simulink model "SG__MDL_IO334"  (R2022b)
settings: Solver=FixedStepAuto  StartTime=0.0  StopTime=Inf  RelTol=1e-3  EnableMultiTasking=on
model workspace (MAT data in the model file):
  a = 0.28
  ff = 1200
  fi = 150
  tmax = 40
libraries: simulink x6, dspsigops x5, hdlsllib x2, slrealtimeloglib x1, SG_library x1, dspsrcs4 x1
settings Model: SimulationMode=external  Creator=padlewsk  LastModifiedBy=padlewsk
settings SolverCC: ConcurrentTasks=on  AlgebraicLoopSolver=TrustRegion  PositivePriorityOrder=on  AutoInsertRateTranBlk=on
settings DataIOCC: SaveFormat=StructureWithTime
settings OptimizationCC: BlockReduction=off  OptimizeBlockIOStorage=off
settings DebuggingCC: TasksWithSamePriorityMsg=none  UnconnectedInputMsg=warning  UnconnectedOutputMsg=warning  UnconnectedLineMsg=warning
settings HardwareCC: ProdBitPerLong=64  ProdLongLongMode=on  ProdHWDeviceType=Intel->x86-64 (Linux 64)
settings ModelReferenceCC: EnableRefExpFcnMdlSchedulingChecks=on
settings RTWCC: Description=Simulink Real-Time  SystemTargetFile=slrealtime.tlc  TemplateMakefile=slrealtime_default_tmf  Toolchain=Simulink Real-Time Toolchain  BuildConfiguration=Faster Runs  CodeExecutionProfiling=on  TargetLang=C++

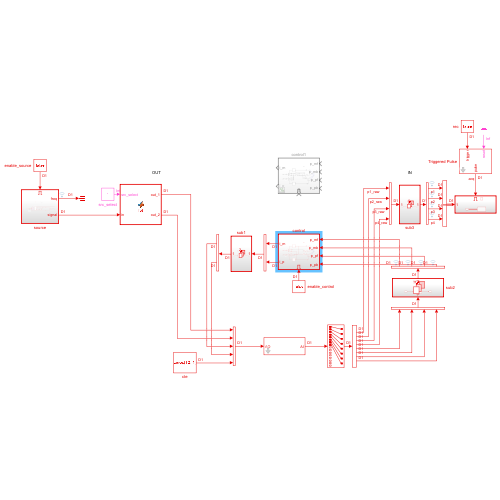
[thumbnail: Simulink's stored preview of the top-level diagram]
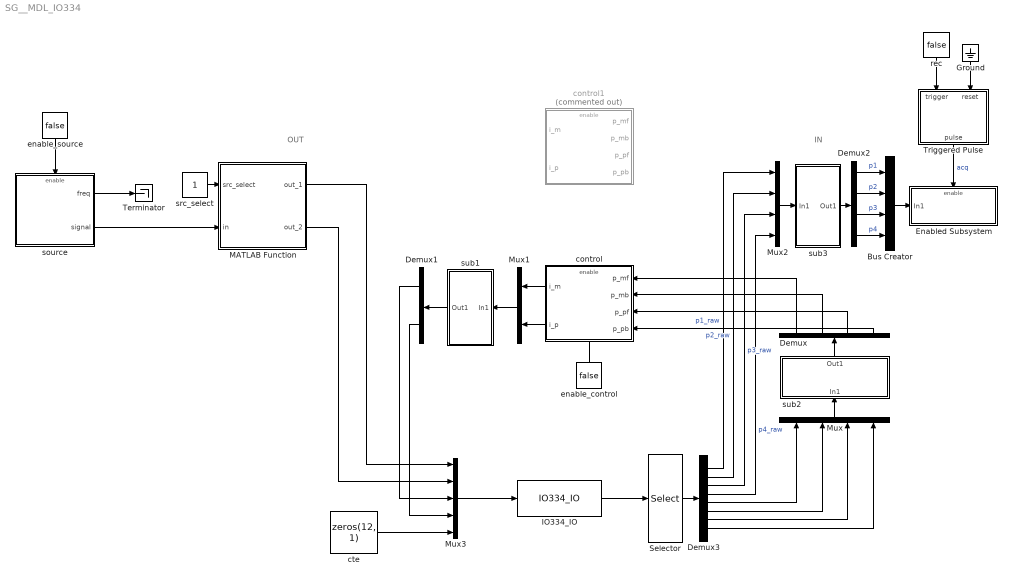
== system SG__MDL_IO334 ==
  note: IN
  note: OUT
  Bus Creator : BusCreator  Inputs=4
  Demux : Demux
  Demux1 : Demux  Outputs=2
  Demux2 : Demux
  Demux3 : Demux  Outputs=8
  Enabled Subsystem : Subsystem  TreatAsAtomicUnit=on
  Ground : Ground
  IO334_IO : SG_library/Built elements/IO334_IO  ts=2.5e-05  OutputRange=Auto (same as ADC)
  MATLAB Function : MATLAB Function  TreatAsAtomicUnit=on
  Mux : Mux
  Mux1 : Mux  Inputs=2
  Mux2 : Mux
  Mux3 : Mux  Inputs=5
  Selector : Selector  InputPortWidth=16  IndexOptions=Index vector (dialog)  Indices=1:8  OutputSizes=1
  Terminator : Terminator
  Triggered Pulse : Subsystem  mask(Triggered Pulse){N=4}
      mask prompts: N "Length (N samples)"
      mask help: Generates a single pulse of N samples length
  control : Subsystem
  control1 : Subsystem  Commented=on
  cte : Constant  Value=zeros(12, 1)  SampleTime=-1
  enable_control : Constant  Value=false  SampleTime=-1
  enable_source : Constant  Value=false  SampleTime=-1
  rec : Constant  Value=false  SampleTime=-1
  source : Subsystem  TreatAsAtomicUnit=on
  src_select : Constant
  sub1 : Subsystem  TreatAsAtomicUnit=on
  sub2 : Subsystem  TreatAsAtomicUnit=on
  sub3 : Subsystem  TreatAsAtomicUnit=on
  wires:
  enable_source/1 -> source/Enable
  Ground/1 -> Triggered Pulse/2(reset)
  rec/1 -> Triggered Pulse/1(trigger)
  Bus Creator/1 -> Enabled Subsystem/1(In1)
  source/1(freq) -> Terminator/1
  source/2(signal) -> MATLAB Function/2(in)
  src_select/1 -> MATLAB Function/1(src_select)
  Mux/1 -> sub2/1(In1)
  sub2/1(Out1) -> Demux/1
  Mux1/1 -> sub1/1(In1)
  sub1/1(Out1) -> Demux1/1
  sub3/1(Out1) -> Demux2/1
  Mux2/1 -> sub3/1(In1)
  Demux3/1 -> Mux2/1  "p1_raw"
  Demux3/2 -> Mux2/2  "p2_raw"
  Demux3/3 -> Mux2/3  "p3_raw"
  Demux3/4 -> Mux2/4  "p4_raw"
  Demux2/2 -> Bus Creator/2  "p2"
  Demux2/1 -> Bus Creator/1  "p1"
  Demux2/3 -> Bus Creator/3  "p3"
  Demux2/4 -> Bus Creator/4  "p4"
  control/1(i_m) -> Mux1/1
  control/2(i_p) -> Mux1/2
  enable_control/1 -> control/Enable
  Demux/1 -> control/1(p_mf)
  Demux/2 -> control/2(p_mb)
  Demux/3 -> control/3(p_pf)
  Demux/4 -> control/4(p_pb)
  IO334_IO/1 -> Selector/1
  Mux3/1 -> IO334_IO/1
  Selector/1 -> Demux3/1
  Demux3/5 -> Mux/1
  Demux3/6 -> Mux/2
  Demux3/7 -> Mux/3
  Demux3/8 -> Mux/4
  cte/1 -> Mux3/5
  Demux1/1 -> Mux3/3
  Demux1/2 -> Mux3/4
  MATLAB Function/2(out_2) -> Mux3/2
  MATLAB Function/1(out_1) -> Mux3/1
  Triggered Pulse/1(pulse) -> Enabled Subsystem/Enable  "acq"

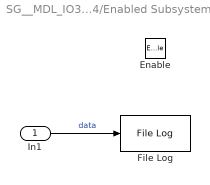
== system SG__MDL_IO334/Enabled Subsystem ==
  In1 : Inport
  Enable : EnablePort
  File Log : slrealtimeloglib/File Log  decimation=1  inputProcessing=Elements as channels (sample based)
  wires:
  In1/1 -> File Log/1  "data"

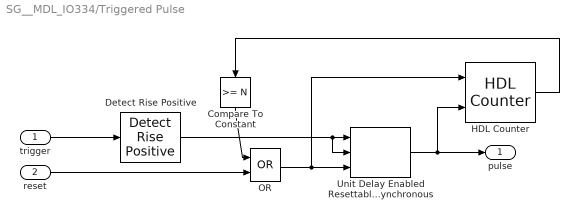
== system SG__MDL_IO334/Triggered Pulse ==
  trigger : Inport
  reset : Inport  Port=2
  Compare To Constant : simulink/Logic and Bit Operations/Compare To Constant  relop=>=  const=N  OutDataTypeStr=boolean
  Detect Rise Positive : simulink/Logic and Bit Operations/Detect Rise Positive  vinit=0  OutDataTypeStr=boolean
  HDL Counter : hdlsllib/Sources/HDL Counter  CountType=Free running  CountInit=1  CountStep=1  CountMax=25  CountFromType=Initial value  CountFrom=1  CountResetPort=on  CountLoadPort=off  CountEnbPort=on  CountDirPort=off  CountHitOutputPort=off  CountDataType=Unsigned  CountWordLen=32  CountFracLen=0  CountSampTime=1
  OR : Logic  Operator=OR  AllPortsSameDT=off  OutDataTypeStr=boolean
  Unit Delay Enabled Resettable Synchronous : hdlsllib/Discrete/Unit Delay Enabled Resettable Synchronous  InitialCondition=0.0  SampleTime=-1
  pulse : Outport  VectorParamsAs1DForOutWhenUnconnected=off
  wires:
  OR/1 -> Unit Delay Enabled Resettable Synchronous/3, HDL Counter/1
  trigger/1 -> Detect Rise Positive/1
  Unit Delay Enabled Resettable Synchronous/1 -> HDL Counter/2, pulse/1
  Compare To Constant/1 -> OR/1
  reset/1 -> OR/2
  Detect Rise Positive/1 -> Unit Delay Enabled Resettable Synchronous/1, Unit Delay Enabled Resettable Synchronous/2
  HDL Counter/1 -> Compare To Constant/1

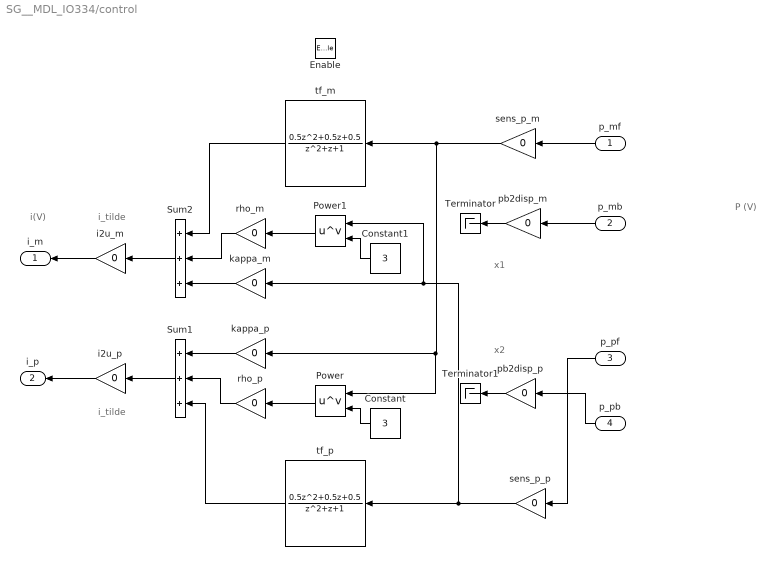
== system SG__MDL_IO334/control ==
  note: x2
  note: P (V)
  note: i_tilde
  note: i(V)
  note: i_tilde
  note: x1
  p_mf : Inport
  p_mb : Inport  Port=2
  p_pf : Inport  Port=3
  p_pb : Inport  Port=4
  Enable : EnablePort
  Constant : Constant  Value=3
  Constant1 : Constant  Value=3
  Power : Math  Operator=pow
  Power1 : Math  Operator=pow
  Sum1 : Sum  Inputs=+++
  Sum2 : Sum  Inputs=+++
  Terminator : Terminator
  Terminator1 : Terminator
  i2u_m : Gain  Gain=0
  i2u_p : Gain  Gain=0
  kappa_m : Gain  Gain=0
  kappa_p : Gain  Gain=0
  pb2disp_m : Gain  Gain=0
  pb2disp_p : Gain  Gain=0
  rho_m : Gain  Gain=0
  rho_p : Gain  Gain=0
  sens_p_m : Gain  Gain=0
  sens_p_p : Gain  Gain=0
  tf_m : DiscreteTransferFcn  Numerator="[0.5         0.5         0.5]"  Denominator="[1  1  1]"
  tf_p : DiscreteTransferFcn  Numerator="[0.5         0.5         0.5]"  Denominator="[1  1  1]"
  i_m : Outport
  i_p : Outport  Port=2
  wires:
  p_mb/1 -> pb2disp_m/1
  p_pb/1 -> pb2disp_p/1
  p_mf/1 -> sens_p_m/1
  sens_p_m/1 -> Power/1, kappa_p/1, tf_m/1
  sens_p_p/1 -> Power1/1, kappa_m/1, tf_p/1
  i2u_m/1 -> i_m/1
  i2u_p/1 -> i_p/1
  rho_p/1 -> Sum1/2
  tf_p/1 -> Sum1/3
  kappa_p/1 -> Sum1/1
  Sum1/1 -> i2u_p/1
  kappa_m/1 -> Sum2/3
  rho_m/1 -> Sum2/2
  tf_m/1 -> Sum2/1
  Sum2/1 -> i2u_m/1
  Power/1 -> rho_p/1
  Constant/1 -> Power/2
  Power1/1 -> rho_m/1
  Constant1/1 -> Power1/2
  pb2disp_m/1 -> Terminator/1
  pb2disp_p/1 -> Terminator1/1
  p_pf/1 -> sens_p_p/1

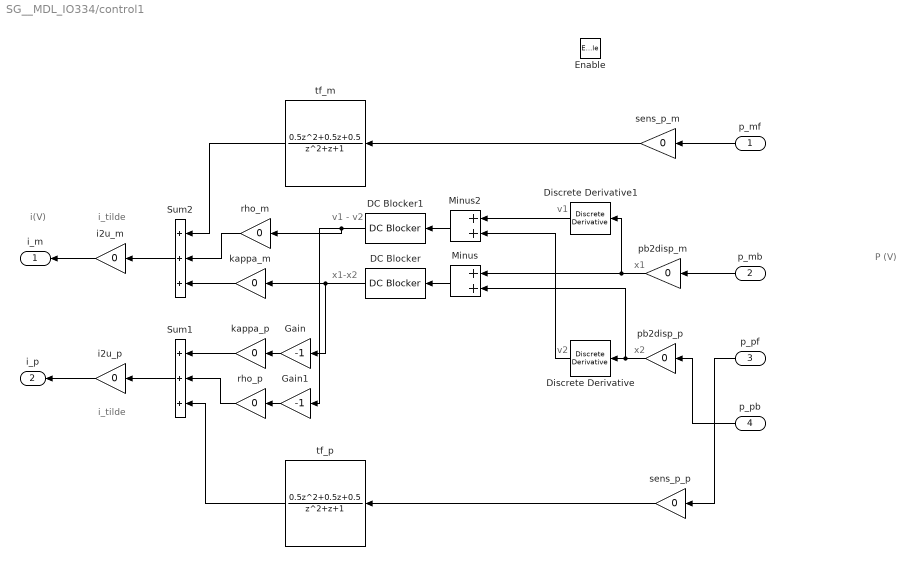
== system SG__MDL_IO334/control1 ==
  note: x2
  note: v2
  note: v1
  note: v1 - v2
  note: P (V)
  note: i_tilde
  note: i(V)
  note: i_tilde
  note: x1-x2
  note: x1
  p_mf : Inport
  p_mb : Inport  Port=2
  p_pf : Inport  Port=3
  p_pb : Inport  Port=4
  Enable : EnablePort
  DC Blocker : dspsigops/DC Blocker  Algorithm=FIR  NormalizedBandwidth=0.001  Length=50  Order=6  SimulateUsing=Code generation
      settings: LibrarySourceBlock=dsphdlsupportsigops/DC Blocker
  DC Blocker1 : dspsigops/DC Blocker  Algorithm=FIR  NormalizedBandwidth=0.001  Length=50  Order=6  SimulateUsing=Code generation
      settings: LibrarySourceBlock=dsphdlsupportsigops/DC Blocker
  Discrete Derivative : simulink/Discrete/Discrete Derivative  gainval=1.0  ICPrevScaledInput=0.0  OutMin=[]  OutMax=[]  OutDataType=fixdt(1, 16)  OutScaling=2^-10  DoSatur=off
  Discrete Derivative1 : simulink/Discrete/Discrete Derivative  gainval=1.0  ICPrevScaledInput=0.0  OutMin=[]  OutMax=[]  OutDataType=fixdt(1, 16)  OutScaling=2^-10  DoSatur=off
  Gain : Gain  Gain=-1
  Gain1 : Gain  Gain=-1
  Minus : Sum
  Minus2 : Sum
  Sum1 : Sum  Inputs=+++
  Sum2 : Sum  Inputs=+++
  i2u_m : Gain  Gain=0
  i2u_p : Gain  Gain=0
  kappa_m : Gain  Gain=0
  kappa_p : Gain  Gain=0
  pb2disp_m : Gain  Gain=0
  pb2disp_p : Gain  Gain=0
  rho_m : Gain  Gain=0
  rho_p : Gain  Gain=0
  sens_p_m : Gain  Gain=0
  sens_p_p : Gain  Gain=0
  tf_m : DiscreteTransferFcn  Numerator="[0.5         0.5         0.5]"  Denominator="[1  1  1]"
  tf_p : DiscreteTransferFcn  Numerator="[0.5         0.5         0.5]"  Denominator="[1  1  1]"
  i_m : Outport
  i_p : Outport  Port=2
  wires:
  p_mb/1 -> pb2disp_m/1
  p_pf/1 -> sens_p_p/1
  p_pb/1 -> pb2disp_p/1
  p_mf/1 -> sens_p_m/1
  sens_p_m/1 -> tf_m/1
  sens_p_p/1 -> tf_p/1
  i2u_m/1 -> i_m/1
  i2u_p/1 -> i_p/1
  pb2disp_m/1 -> Discrete Derivative1/1, Minus/1
  Minus2/1 -> DC Blocker1/1
  Minus/1 -> DC Blocker/1
  DC Blocker/1 -> Gain/1, kappa_m/1
  rho_p/1 -> Sum1/2
  tf_p/1 -> Sum1/3
  kappa_p/1 -> Sum1/1
  Sum1/1 -> i2u_p/1
  kappa_m/1 -> Sum2/3
  rho_m/1 -> Sum2/2
  Discrete Derivative1/1 -> Minus2/1
  tf_m/1 -> Sum2/1
  Sum2/1 -> i2u_m/1
  DC Blocker1/1 -> Gain1/1, rho_m/1
  Discrete Derivative/1 -> Minus2/2
  pb2disp_p/1 -> Minus/2, Discrete Derivative/1
  Gain/1 -> kappa_p/1
  Gain1/1 -> rho_p/1

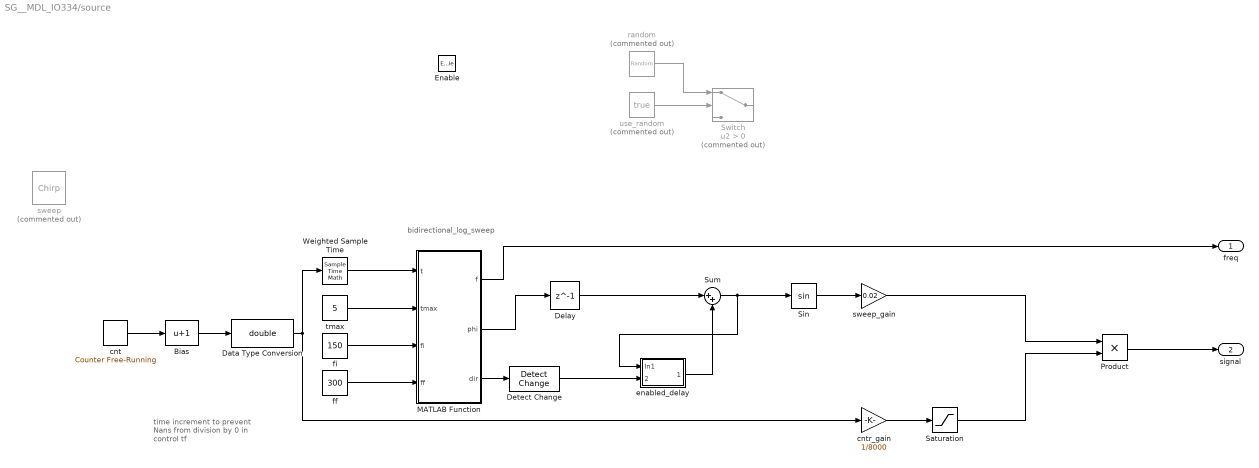
== system SG__MDL_IO334/source ==
  note: bidirectional_log_sweep
  note: time increment to prevent Nans from division by 0 in control tf
  Enable : EnablePort  StatesWhenEnabling=reset
  Bias : Bias  Bias=1  SaturateOnIntegerOverflow=off
  Data Type Conversion : DataTypeConversion  OutDataTypeStr=double  SaturateOnIntegerOverflow=off  RndMeth=Floor
  Delay : Delay  DelayLength=1
  Detect Change : simulink/Logic and Bit Operations/Detect Change  vinit=false  OutDataTypeStr=boolean
  MATLAB Function : MATLAB Function  TreatAsAtomicUnit=on
  Product : Product
  Saturation : Saturate  UpperLimit=1  LowerLimit=0
  Sin : Trigonometry
  Sum : Sum  Inputs=|++
  Switch : Switch  Commented=on  Criteria=u2 > Threshold  SaturateOnIntegerOverflow=off  InputSameDT=off
  Weighted Sample Time : SampleTimeMath  TsampMathOp=*
  cnt : simulink/Sources/Counter Free-Running  NumBits=32  tsamp=-1
  cntr_gain : Gain  Gain=1/8000  ParamDataTypeStr=double
  enabled_delay : Subsystem
  ff : Constant  Value=300
  fi : Constant  Value=150
  random : RandomNumber  Commented=on  Variance=0.5  SampleTime=3.5e-05
  sweep : dspsrcs4/Chirp  Commented=on  sweep=Logarithmic  mode=Bidirectional  f0=150  f1=1200  t1=10  Tsweep=20  phase=0  Ts=3.5e-05  spf=1  datatype=Double  OutputFrames=off
  sweep_gain : Gain  Gain=0.02
  tmax : Constant  Value=5
  use_random : Constant  Commented=on  Value=true  SampleTime=-1
  freq : Outport  OutputWhenDisabled=reset  InitialOutput=0  VectorParamsAs1DForOutWhenUnconnected=off
  signal : Outport  Port=2  OutputWhenDisabled=reset  InitialOutput=0  VectorParamsAs1DForOutWhenUnconnected=off
  wires:
  use_random/1 -> Switch/2
  random/1 -> Switch/1
  sweep_gain/1 -> Product/1
  cntr_gain/1 -> Saturation/1
  Product/1 -> signal/1
  MATLAB Function/2(phi) -> Delay/1
  Saturation/1 -> Product/2
  Weighted Sample Time/1 -> MATLAB Function/1(t)
  Data Type Conversion/1 -> cntr_gain/1, Weighted Sample Time/1
  MATLAB Function/1(f) -> freq/1
  Sin/1 -> sweep_gain/1
  MATLAB Function/3(dir) -> Detect Change/1
  Detect Change/1 -> enabled_delay/2(enable)
  Delay/1 -> Sum/1
  enabled_delay/1(Out1) -> Sum/2
  Sum/1 -> enabled_delay/1(In1), Sin/1
  cnt/1 -> Bias/1
  Bias/1 -> Data Type Conversion/1
  ff/1 -> MATLAB Function/4(ff)
  tmax/1 -> MATLAB Function/2(tmax)
  fi/1 -> MATLAB Function/3(fi)

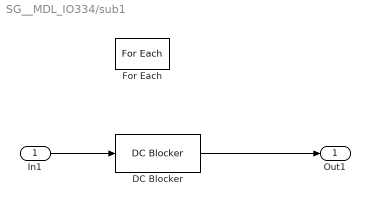
== system SG__MDL_IO334/sub1 ==
  In1 : Inport  Partition=on  PartitionDimension=1  PartitionWidth=1  PartitionOffset=0
  DC Blocker : dspsigops/DC Blocker  Algorithm=FIR  NormalizedBandwidth=0.001  Length=50  Order=6  SimulateUsing=Code generation
      settings: LibrarySourceBlock=dsphdlsupportsigops/DC Blocker
  For Each : ForEach  DisableCoverage=on
  Out1 : Outport  ConcatenationDimension=1
  wires:
  In1/1 -> DC Blocker/1
  DC Blocker/1 -> Out1/1

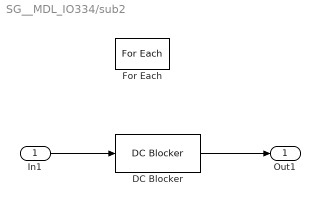
== system SG__MDL_IO334/sub2 ==
  In1 : Inport  Partition=on  PartitionDimension=1  PartitionWidth=1  PartitionOffset=0
  DC Blocker : dspsigops/DC Blocker  Algorithm=FIR  NormalizedBandwidth=0.001  Length=50  Order=6  SimulateUsing=Code generation
      settings: LibrarySourceBlock=dsphdlsupportsigops/DC Blocker
  For Each : ForEach  DisableCoverage=on
  Out1 : Outport  ConcatenationDimension=1
  wires:
  In1/1 -> DC Blocker/1
  DC Blocker/1 -> Out1/1

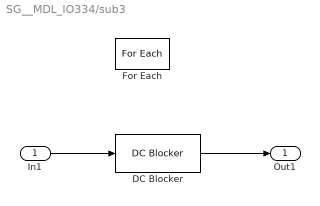
== system SG__MDL_IO334/sub3 ==
  In1 : Inport  Partition=on  PartitionDimension=1  PartitionWidth=1  PartitionOffset=0
  DC Blocker : dspsigops/DC Blocker  Algorithm=FIR  NormalizedBandwidth=0.001  Length=50  Order=6  SimulateUsing=Code generation
      settings: LibrarySourceBlock=dsphdlsupportsigops/DC Blocker
  For Each : ForEach  DisableCoverage=on
  Out1 : Outport  ConcatenationDimension=1
  wires:
  In1/1 -> DC Blocker/1
  DC Blocker/1 -> Out1/1

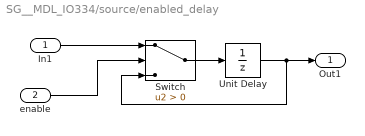
== system SG__MDL_IO334/source/enabled_delay ==
  In1 : Inport
  enable : Inport  Port=2
  Switch : Switch  Criteria=u2 > Threshold  SaturateOnIntegerOverflow=off  InputSameDT=off
  Unit Delay : UnitDelay  SampleTime=-1  HasFrameUpgradeWarning=on
  Out1 : Outport
  wires:
  Unit Delay/1 -> Switch/3, Out1/1
  Switch/1 -> Unit Delay/1
  In1/1 -> Switch/1
  enable/1 -> Switch/2

== matlab function SG__MDL_IO334/MATLAB Function ==
  data: src_select input; in input; out_1 output; out_2 output
function [out_1, out_2] = fct(src_select, in)
out_1 = 0;
out_2 = 0;
if src_select == 1
    out_1 = in;
elseif src_select == 2
    out_2 = in;
end

== matlab function SG__MDL_IO334/source/MATLAB Function ==
  data: f output; t input; tmax input; phi output; dir output; fi input; ff input
function [f, phi, dir] = fcn(t, tmax, fi, ff)
%tmax is the time at which the maximum frequency is reached

t = mod(t, 2*tmax);

if t < tmax
    % up
    dir = 1;
    
    
    % linear (CF wikipedia)
%     phi = 2*pi*(0.5*(ff - fi)*t^2/tmax + fi*t);
%     f = fi + (ff - fi)*t/tmax;
    
    % logarithmic %%% https://en.wikipedia.org/wiki/Chirp
    k = log((ff/fi)^(1/tmax));
    phi = 2*pi*fi*(exp(k*t) - 1)/k;
    f = fi*exp(k*t);
else
    % down
    dir = -1;
    
    
    % linear (CF wikipedia)
%     phi = 2*pi*(0.5*(fi - ff)*(t-tmax)^2/tmax + ff*(t-tmax)); % linear
%     f = ff + (fi - ff)*(t - tmax)/tmax;
    
    % logarithmic
    k = log((fi/ff)^(1/tmax));
    phi = 2*pi*ff*(exp(k*(t - tmax)) - 1)/k;
    f = ff*exp(k*(t-tmax));
end

phi = mod(phi, 2*pi);
